simulink model "H637"  (Simulink 7.7)
settings: Solver=ode45  StartTime=0.0  StopTime=7.0  RelTol=1e-5
libraries: simulink x7
settings Model: Creator=Admin  LastModifiedBy=Admin

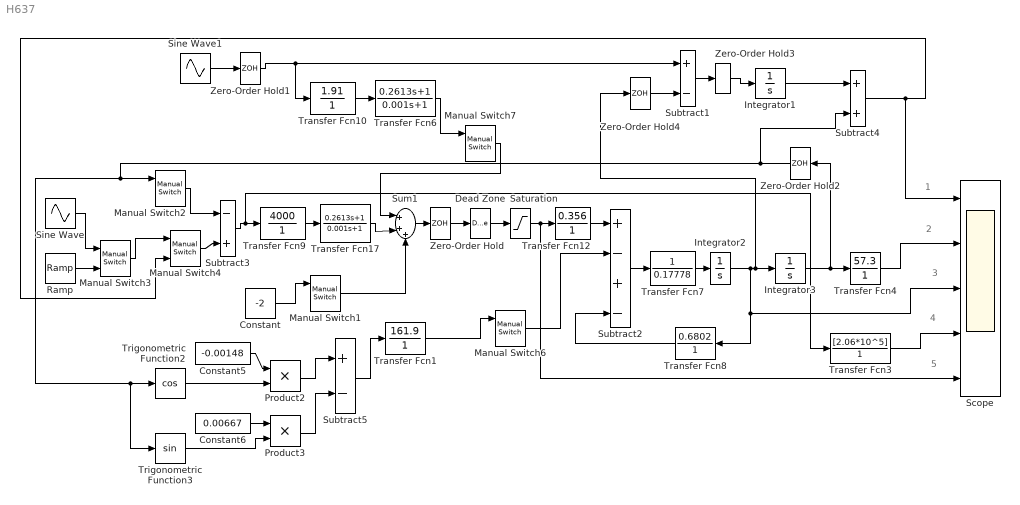
== system H637 ==
  note: 1
  note: 2
  note: 3
  note: 4
  note: 5
  Constant : Constant  Value=-2
  Constant5 : Constant  Value=-0.00148
  Constant6 : Constant  Value=0.00667
  Dead Zone : DeadZone  LowerValue=-1.4  UpperValue=1.4  SaturateOnIntegerOverflow=on
  Integrator1 : Integrator
  Integrator2 : Integrator
  Integrator3 : Integrator
  Manual Switch{1..3,6..7} (5 alike) : simulink/Signal Routing/Manual Switch  SystemSampleTime=-1  sw=1  action=0  varsize=off
  Manual Switch4 : simulink/Signal Routing/Manual Switch  SystemSampleTime=-1  sw=0  action=0  varsize=off
  Product2 : Product  RndMeth=Zero
  Product3 : Product  RndMeth=Zero
  Ramp : simulink/Sources/Ramp  SystemSampleTime=-1  slope=1  start=0  X0=0
  Saturation : Saturate  UpperLimit=27  LowerLimit=-27
  Scope : Scope  NumInputPorts=5
      settings: TimeRange=5  YMin=-30~-500~-1.5~-30~-500  YMax=30~2500~1.5~30~2500  MaxDataPoints=5000000
  Sine Wave : Sin  Amplitude=0.5  Frequency=2  SampleTime=0
  Sine Wave1 : Sin  Frequency=2  Phase=1.57  SampleTime=0
  Subtract1 : Sum  Inputs=+-
  Subtract2 : Sum  Inputs=+-+-
  Subtract3 : Sum  Inputs=-+
  Subtract4 : Sum
  Subtract5 : Sum  Inputs=+-
  Sum1 : Sum  Inputs=|+++
  Transfer Fcn1 : TransferFcn  Numerator=[161.9]  Denominator=[ 1 ]
  Transfer Fcn10 : TransferFcn  Numerator=1.91  Denominator=[ 1 ]
  Transfer Fcn12 : TransferFcn  Numerator=[0.356]  Denominator=[ 1 ]
  Transfer Fcn17 : TransferFcn  Numerator=[0.2613 1]  Denominator=[0.001 1]
  Transfer Fcn3 : TransferFcn  Numerator=[2.06*10^5]  Denominator=[ 1 ]
  Transfer Fcn4 : TransferFcn  Numerator=[57.3]  Denominator=[ 1 ]
  Transfer Fcn6 : TransferFcn  Numerator=[0.2613 1]  Denominator=[0.001 1]
  Transfer Fcn7 : TransferFcn  Denominator=0.17778
  Transfer Fcn8 : TransferFcn  Numerator=[0.6802]  Denominator=[ 1]
  Transfer Fcn9 : TransferFcn  Numerator=4000  Denominator=[ 1 ]
  Trigonometric Function2 : Trigonometry  Operator=cos
  Trigonometric Function3 : Trigonometry
  Zero-Order Hold : ZeroOrderHold  SampleTime=1/19531.25
  Zero-Order Hold1 : ZeroOrderHold  SampleTime=1/39062.5
  Zero-Order Hold2 : ZeroOrderHold  SampleTime=1/25000
  Zero-Order Hold3 : ZeroOrderHold  SampleTime=1/1000
  Zero-Order Hold4 : ZeroOrderHold  SampleTime=1/25000
  wires:
  Subtract2/1 -> Transfer Fcn7/1
  Integrator2/1 -> Integrator3/1, Zero-Order Hold4/1, Transfer Fcn8/1, Scope/3
  Transfer Fcn7/1 -> Integrator2/1
  Integrator3/1 -> Transfer Fcn4/1, Zero-Order Hold2/1
  Subtract3/1 -> Transfer Fcn9/1, Transfer Fcn3/1
  Transfer Fcn8/1 -> Subtract2/4
  Transfer Fcn12/1 -> Subtract2/1
  Transfer Fcn9/1 -> Transfer Fcn17/1
  Constant5/1 -> Product2/1
  Trigonometric Function2/1 -> Product2/2
  Constant6/1 -> Product3/1
  Trigonometric Function3/1 -> Product3/2
  Product3/1 -> Subtract5/2
  Product2/1 -> Subtract5/1
  Subtract5/1 -> Transfer Fcn1/1
  Manual Switch6/1 -> Subtract2/2
  Transfer Fcn1/1 -> Manual Switch6/1
  Constant/1 -> Manual Switch1/1
  Manual Switch2/1 -> Subtract3/1
  Saturation/1 -> Transfer Fcn12/1, Scope/5
  Zero-Order Hold/1 -> Dead Zone/1
  Sum1/1 -> Zero-Order Hold/1
  Sine Wave/1 -> Manual Switch3/1
  Ramp/1 -> Manual Switch3/2
  Manual Switch4/1 -> Subtract3/2
  Manual Switch3/1 -> Manual Switch4/1
  Subtract1/1 -> Zero-Order Hold3/1
  Sine Wave1/1 -> Zero-Order Hold1/1
  Integrator1/1 -> Subtract4/1
  Subtract4/1 -> Manual Switch4/2, Scope/1
  Zero-Order Hold3/1 -> Integrator1/1
  Transfer Fcn10/1 -> Transfer Fcn6/1
  Manual Switch1/1 -> Sum1/3
  Transfer Fcn17/1 -> Sum1/2
  Zero-Order Hold1/1 -> Transfer Fcn10/1, Subtract1/1
  Transfer Fcn6/1 -> Manual Switch7/1
  Manual Switch7/1 -> Sum1/1
  Transfer Fcn4/1 -> Scope/2
  Transfer Fcn3/1 -> Scope/4
  Zero-Order Hold4/1 -> Subtract1/2
  Zero-Order Hold2/1 -> Trigonometric Function2/1, Trigonometric Function3/1, Manual Switch2/1, Subtract4/2
  Dead Zone/1 -> Saturation/1
